simulink model "p2_2"  (R2022b)
settings: Solver=VariableStepAuto  StartTime=0.0  StopTime=20.0  RelTol=1e-3
model workspace (MAT data in the model file):
  B = Simulink.Parameter
  B.DataType = 'auto'
  B.Complexity = 'real'
  B.Dimensions = [0 0]
settings Model: Creator=Ausu  LastModifiedBy=Ausu

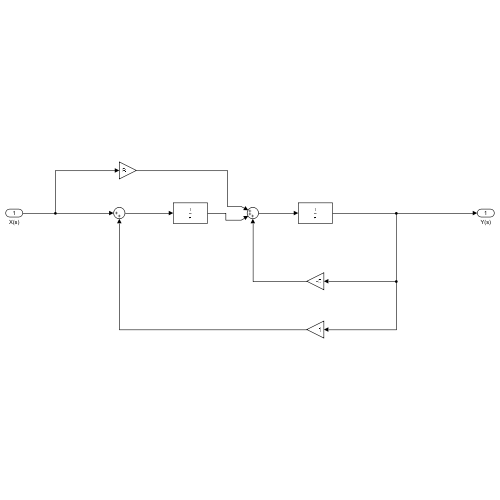
[thumbnail: Simulink's stored preview of the top-level diagram]
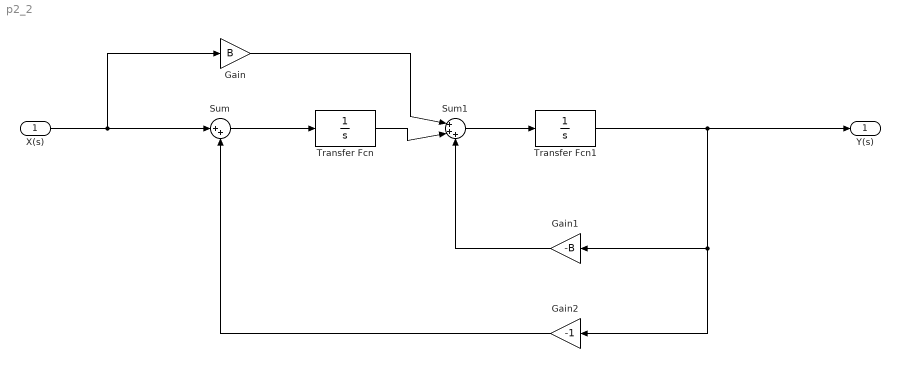
== system p2_2 ==
  X(s) : Inport
  Gain : Gain  Gain=B
  Gain1 : Gain  Gain=-B
  Gain2 : Gain  Gain=-1
  Sum : Sum  Inputs=|++
  Sum1 : Sum  Inputs=|+++
  Transfer Fcn : TransferFcn  Denominator=[1 0]
  Transfer Fcn1 : TransferFcn  Denominator=[1 0]
  Y(s) : Outport
  wires:
  X(s)/1 -> Gain/1, Sum/1
  Sum/1 -> Transfer Fcn/1
  Transfer Fcn/1 -> Sum1/2
  Gain/1 -> Sum1/1
  Sum1/1 -> Transfer Fcn1/1
  Transfer Fcn1/1 -> Gain2/1, Gain1/1, Y(s)/1
  Gain1/1 -> Sum1/3
  Gain2/1 -> Sum/2
